simulink library "bts"  (Simulink 8.1)
settings: Solver=ode1  StartTime=0.0  StopTime=Inf  FixedStep=0.001  RelTol=1e-3
PostLoadFcn:
  | , if any(exist('dsrtsu_mdlpostloadfcn', 'file') == [2, 3, 6]), try dsrtsu_mdlpostloadfcn('Execute', bdroot); catch fprintf('Error in PostLoadFcn (dsrtsu_mdlpostloadfcn) for model "%s":\n %s\n', bdroot, lasterr); end, end,
undefined symbols (not defined in the file or in its folder): KACC_BTSTargetBrakingSpd_kph, KACC_BTSTargetNoBrakingSpd_kph
libraries: hcu_lib x2
settings Model: DSRTSU_INTERNAL_RTI_VER=450  DSRTSU_INTERNAL_RTI_TYPE=rti1401  RTICANMMDATA=struct('GeneralSetupData',struct('modelroot','D:\ELN150201_TAIWAN\trunk\AdasDragon\software\sw_development\arch\app\acc','generalsettings',struct('filesettings',struct('destfolder',struct('Name','RTICANMM_FILES','Check',1),'buildfolder',struct('Name','.','Check',1),'AbsDestfolder',struct('Name','D:\ELN150201_TAIWAN\trunk\AdasDragon\software\sw_development\arch\app\acc\RTICANMM_FILES'),'AbsBuildfolder',struct('Name','D:\ELN150201_TAIWAN\trunk\AdasDragon\software\sw_development\arch\app\acc'))),'options',struct('addpaths',1,'rmpaths',1,'addtrcexclusion',logical(1),'cannavigator',struct('checkmonitoring',0),'show_usrtrc',0,'use_usrtrc',0),'advanced',struct('options',[1 1 1 1 1 1 1 1 1 1 1 1 1 1 1 1 1 1 1 1 1 1 1 1 1 1 1 1 1 1 1 1 1 1 1 1 1 1 1 1 1 1 1 1 1 1 1 1 1 1 1 1 1 1 1 1 1 1 1 1 1 1 1 1 1 1 1 1 1 1 1 1 1 1 1 1 1 1 1 1 1 1 1 1 1 1 1 1 1 1 1 1 1 1 1 1 1 1 1 1]),'MPSetup',{{}},'modelname','bts','block','bts'))  DSRTSU_INTERNAL_RTIFPGA=40  Creator=AT015411  LastModifiedBy=AT015555

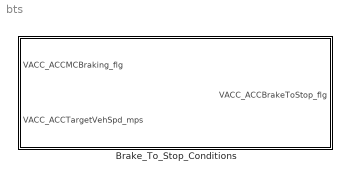
== system bts ==
  Brake_To_Stop_Conditions : Subsystem

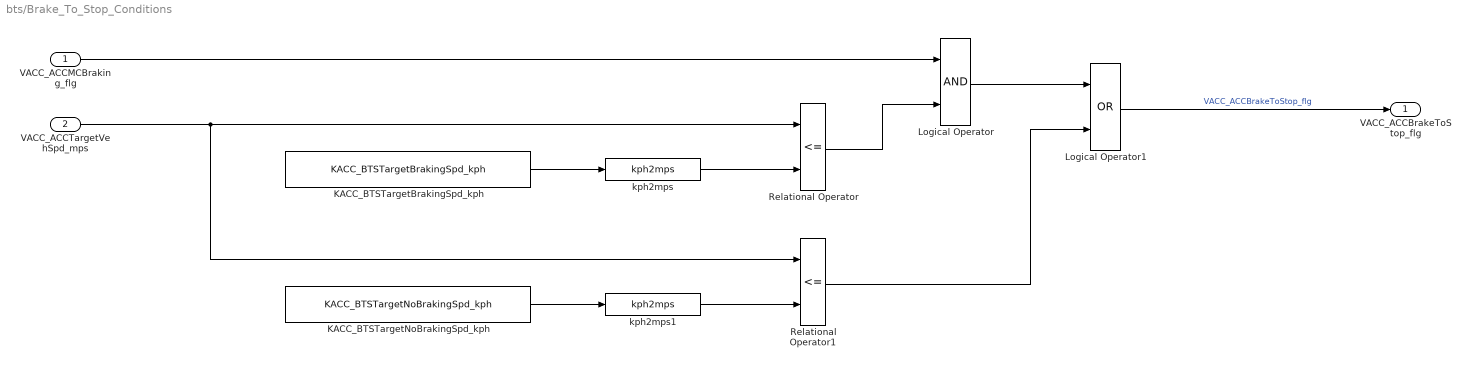
== system bts/Brake_To_Stop_Conditions ==
  VACC_ACCMCBraking_flg : Inport
  VACC_ACCTargetVehSpd_mps : Inport  Port=2
  KACC_BTSTargetBrakingSpd_kph : Constant  Value=KACC_BTSTargetBrakingSpd_kph
  KACC_BTSTargetNoBrakingSpd_kph : Constant  Value=KACC_BTSTargetNoBrakingSpd_kph
  Logical Operator : Logic  AllPortsSameDT=off  OutDataTypeStr=boolean
  Logical Operator1 : Logic  Operator=OR  AllPortsSameDT=off  OutDataTypeStr=boolean
  Relational Operator : RelationalOperator  Operator=<=  OutDataTypeStr=boolean
  Relational Operator1 : RelationalOperator  Operator=<=  OutDataTypeStr=boolean
  kph2mps : hcu_lib/kph2mps
  kph2mps1 : hcu_lib/kph2mps
  VACC_ACCBrakeToStop_flg : Outport
  wires:
  Logical Operator1/1 -> VACC_ACCBrakeToStop_flg/1  "VACC_ACCBrakeToStop_flg"
  Relational Operator1/1 -> Logical Operator1/2
  Logical Operator/1 -> Logical Operator1/1
  Relational Operator/1 -> Logical Operator/2
  kph2mps1/1 -> Relational Operator1/2
  KACC_BTSTargetNoBrakingSpd_kph/1 -> kph2mps1/1
  VACC_ACCTargetVehSpd_mps/1 -> Relational Operator/1, Relational Operator1/1
  VACC_ACCMCBraking_flg/1 -> Logical Operator/1
  KACC_BTSTargetBrakingSpd_kph/1 -> kph2mps/1
  kph2mps/1 -> Relational Operator/2
